simulink model "baseline_super_ground"  (R2021a)
settings: Solver=FixedStepAuto  StartTime=0.0  StopTime=50  FixedStep=framePeriod_s  RelTol=1e-3
undefined symbols (not defined in the file or in its folder): Aircraft, DiscIntNeverNeededParam, framePeriod_s
libraries: simulink x36
(part 2 of 2)

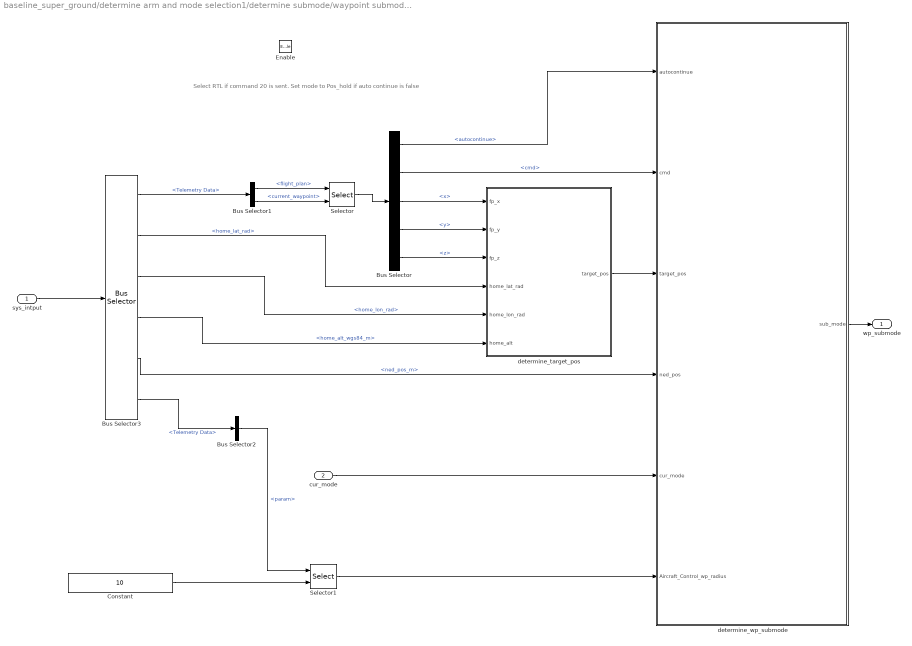
== system baseline_super_ground/determine arm and mode selection1/determine submode/waypoint submodes ==
  note: Select RTL if command 20 is sent. Set mode to Pos_hold if auto continue is false
  sys_intput : Inport
  cur_mode : Inport  Port=2
  Enable : EnablePort
  Bus Selector : BusSelector  OutputSignals=autocontinue,cmd,x,y,z
  Bus Selector1 : BusSelector  OutputSignals=flight_plan,current_waypoint
  Bus Selector2 : BusSelector  OutputSignals=param
  Bus Selector3 : BusSelector  OutputSignals=Telemetry Data,Navigation Filter Data.home_lat_rad,Navigation Filter Data.home_lon_rad,Navigation Filter Data.home_alt_wgs84_m,Navigation Filter Data.ned_pos_m,Telemetry Data
  Constant : Constant  Value=10  OutDataTypeStr=single
  Selector : Selector  IndexMode=Zero-based  InputPortWidth=500  IndexOptions=Index vector (port)  Indices=7  OutputSizes=1
  Selector1 : Selector  IndexMode=Zero-based  IndexOptions=Index vector (port)  Indices=[1 3]  OutputSizes=1
  determine_target_pos : MATLAB Function  TreatAsAtomicUnit=on
  determine_wp_submode : MATLAB Function  TreatAsAtomicUnit=on
  wp_submode : Outport
  wires:
  sys_intput/1 -> Bus Selector3/1
  determine_wp_submode/1(sub_mode) -> wp_submode/1
  Bus Selector3/5 -> determine_wp_submode/4(ned_pos)  "<ned_pos_m>"
  Bus Selector3/2 -> determine_target_pos/4(home_lat_rad)  "<home_lat_rad>"
  Bus Selector3/3 -> determine_target_pos/5(home_lon_rad)  "<home_lon_rad>"
  Bus Selector3/4 -> determine_target_pos/6(home_alt)  "<home_alt_wgs84_m>"
  determine_target_pos/1(target_pos) -> determine_wp_submode/3(target_pos)
  cur_mode/1 -> determine_wp_submode/5(cur_mode)
  Selector1/1 -> determine_wp_submode/6(Aircraft_Control_wp_radius)
  Bus Selector3/1 -> Bus Selector1/1  "<Telemetry Data>"
  Bus Selector1/1 -> Selector/1  "<flight_plan>"
  Bus Selector1/2 -> Selector/2  "<current_waypoint>"
  Selector/1 -> Bus Selector/1
  Bus Selector/2 -> determine_wp_submode/2(cmd)  "<cmd>"
  Bus Selector/1 -> determine_wp_submode/1(autocontinue)  "<autocontinue>"
  Bus Selector/3 -> determine_target_pos/1(fp_x)  "<x>"
  Bus Selector/4 -> determine_target_pos/2(fp_y)  "<y>"
  Bus Selector/5 -> determine_target_pos/3(fp_z)  "<z>"
  Bus Selector3/6 -> Bus Selector2/1  "<Telemetry Data>"
  Constant/1 -> Selector1/2
  Bus Selector2/1 -> Selector1/1  "<param>"

== system baseline_super_ground/Mode Management System/Failsafe_management/Battery failsafe/disarm motor ==
  Enable : EnablePort  StatesWhenEnabling=reset
  Compare To Constant2 : simulink/Logic and Bit Operations/Compare To Constant  relop=>  const=15  OutDataTypeStr=boolean
  Constant : Constant  Value=framePeriod_s
  Sum : Sum  Inputs=|++
  Unit Delay : UnitDelay  SampleTime=-1  HasFrameUpgradeWarning=on
  battery_low_trigger : Outport
  wires:
  Compare To Constant2/1 -> battery_low_trigger/1
  Sum/1 -> Compare To Constant2/1, Unit Delay/1
  Unit Delay/1 -> Sum/2
  Constant/1 -> Sum/1

== system baseline_super_ground/determine arm and mode selection1/Failsafe_management/Battery failsafe/disarm motor ==
  Enable : EnablePort  StatesWhenEnabling=reset
  Compare To Constant2 : simulink/Logic and Bit Operations/Compare To Constant  relop=>  const=15  OutDataTypeStr=boolean
  Constant : Constant  Value=framePeriod_s
  Sum : Sum  Inputs=|++
  Unit Delay : UnitDelay  SampleTime=-1  HasFrameUpgradeWarning=on
  battery_low_trigger : Outport
  wires:
  Compare To Constant2/1 -> battery_low_trigger/1
  Sum/1 -> Compare To Constant2/1, Unit Delay/1
  Unit Delay/1 -> Sum/2
  Constant/1 -> Sum/1

== matlab function baseline_super_ground/command selection/rtl_norm/remap ==
  data: raw_in input; norm_out output; in_min input; in_max input; out_min input; out_max input
function norm_out = remap(raw_in,in_min,in_max,out_min,out_max)
norm_out = (raw_in - in_min) * (out_max - out_min)/(in_max-in_min) + out_min;

== matlab function baseline_super_ground/determine arm and mode selection1/determine submode/rtl submodes/determine_fast_rtl_mode ==
  data: target_pos input; sub_mode output; ned_pos input; cur_mode input; Aircraft_Control_wp_radius input
function sub_mode = determine_fast_rtl(target_pos, ned_pos, cur_mode, Aircraft_Control_wp_radius)

sub_mode = cur_mode;
diff = target_pos(1:2) - ned_pos(1:2);
if norm(diff) <= Aircraft_Control_wp_radius
    sub_mode = int8(4); % land
end

end

== matlab function baseline_super_ground/determine arm and mode selection1/determine submode/waypoint submodes/determine_target_pos ==
  data: fp_x input; target_pos output single size=3; fp_y input; fp_z input; home_lat_rad input; home_lon_rad input; home_alt input
function target_pos = determine_target_pos(fp_x, fp_y, fp_z, home_lat_rad, home_lon_rad, home_alt)


% target_pos = flight_plan_to_ned(flight_plan, cur_wp, home_lat_rad, home_lon_rad, home_alt);

target_pos = mission_item_to_ned(fp_x, fp_y, fp_z, home_lat_rad, home_lon_rad, home_alt);

end

== matlab function baseline_super_ground/command selection/throttle_norm/remap ==
  data: raw_in input; norm_out output; in_min input; in_max input; out_min input; out_max input
function norm_out = remap(raw_in,in_min,in_max,out_min,out_max)
norm_out = (raw_in - in_min) * (out_max - out_min)/(in_max-in_min) + out_min;

== matlab function baseline_super_ground/determine arm and mode selection1/determine submode/waypoint submodes/determine_wp_submode ==
  data: autocontinue input; cmd input; sub_mode output int8; target_pos input; ned_pos input; cur_mode input; Aircraft_Control_wp_radius input size=1
function sub_mode = determine_wp_submode(autocontinue, cmd, target_pos, ned_pos, cur_mode, Aircraft_Control_wp_radius)
% Sub mode select RTL if mission command 20 is reached in the flight plan
% Sub mode select Pos_Hold if auto continued is false

sub_mode = cur_mode;

if cmd == 20
    sub_mode = int8(3); % RTL
    
elseif cmd == 16
    diff = target_pos(1:2) - ned_pos(1:2);
    reached_wp = norm(diff) <= Aircraft_Control_wp_radius;
    if cur_mode ~= 3 && reached_wp && ~autocontinue
        sub_mode = int8(1); % pos hold
    end
end

end

== matlab function baseline_super_ground/cmd to raw pwm1/engine_PWM_denormalize/remap ==
  data: norm_in input; raw_out output; in_min input; in_max input; out_min input; out_max input
function raw_out = remap(norm_in,in_min,in_max,out_min,out_max)
raw_out = (norm_in - in_min) * (out_max - out_min)/(in_max-in_min) + out_min;

== matlab function baseline_super_ground/cmd to raw pwm1/motor_PWM_denormalize/remap ==
  data: norm_in input; raw_out output; in_min input; in_max input; out_min input; out_max input
function raw_out = remap(norm_in,in_min,in_max,out_min,out_max)
raw_out = (norm_in - in_min) * (out_max - out_min)/(in_max-in_min) + out_min;

== matlab function baseline_super_ground/command selection/pitch_norm/remap ==
  data: raw_in input; norm_out output; in_min input; in_max input; out_min input; out_max input
function norm_out = remap(raw_in,in_min,in_max,out_min,out_max)
norm_out = (raw_in - in_min) * (out_max - out_min)/(in_max-in_min) + out_min;

== matlab function baseline_super_ground/command selection/roll_norm/remap ==
  data: raw_in input; norm_out output; in_min input; in_max input; out_min input; out_max input
function norm_out = remap(raw_in,in_min,in_max,out_min,out_max)
norm_out = (raw_in - in_min) * (out_max - out_min)/(in_max-in_min) + out_min;

== matlab function baseline_super_ground/command selection/yaw_norm/remap ==
  data: raw_in input; norm_out output; in_min input; in_max input; out_min input; out_max input
function norm_out = remap(raw_in,in_min,in_max,out_min,out_max)
norm_out = (raw_in - in_min) * (out_max - out_min)/(in_max-in_min) + out_min;

== matlab function baseline_super_ground/command selection/e_stop_norm/remap ==
  data: raw_in input; norm_out output; in_min input; in_max input; out_min input; out_max input
function norm_out = remap(raw_in,in_min,in_max,out_min,out_max)
norm_out = (raw_in - in_min) * (out_max - out_min)/(in_max-in_min) + out_min;

== matlab function baseline_super_ground/command selection/mode_norm/remap ==
  data: raw_in input; norm_out output; in_min input; in_max input; out_min input; out_max input
function norm_out = remap(raw_in,in_min,in_max,out_min,out_max)
norm_out = (raw_in - in_min) * (out_max - out_min)/(in_max-in_min) + out_min;

== matlab function baseline_super_ground/command selection/engine_cmd_norm/remap ==
  data: raw_in input; norm_out output; in_min input; in_max input; out_min input; out_max input
function norm_out = remap(raw_in,in_min,in_max,out_min,out_max)
norm_out = (raw_in - in_min) * (out_max - out_min)/(in_max-in_min) + out_min;

== matlab function baseline_super_ground/command selection/relay_norm/remap ==
  data: raw_in input; norm_out output; in_min input; in_max input; out_min input; out_max input
function norm_out = remap(raw_in,in_min,in_max,out_min,out_max)
norm_out = (raw_in - in_min) * (out_max - out_min)/(in_max-in_min) + out_min;
